simulink model "second_order_controllar"  (R2024b)
settings: Solver=FixedStepAuto  StartTime=0.0  StopTime=10.0  FixedStep=0.001  RelTol=1e-3
libraries: simulink x1
settings Model: Creator=elija  LastModifiedBy=elija

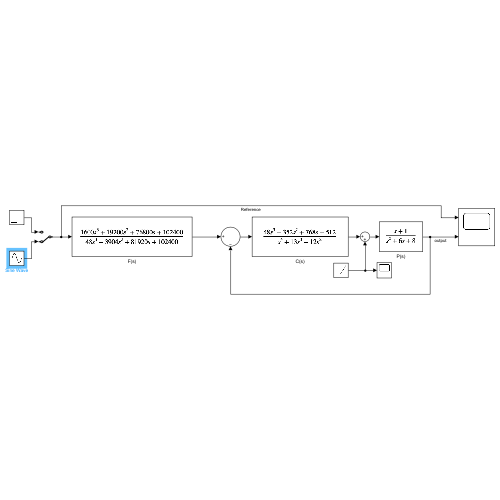
[thumbnail: Simulink's stored preview of the top-level diagram]
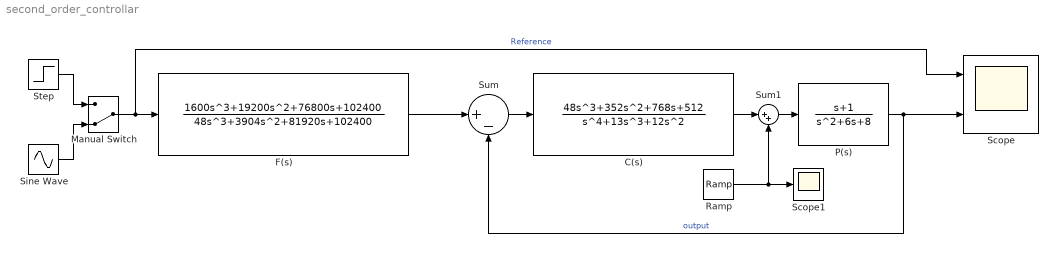
== system second_order_controllar ==
  C(s) : TransferFcn  Numerator=[48 352 768 512]  Denominator=[1 13 12 0 0]
  F(s) : TransferFcn  Numerator=[1600 19200 76800 102400]  Denominator=[48 3904 81920 102400]
  Manual Switch : ManualSwitch  CurrentSetting=0
  P(s) : TransferFcn  Numerator=[1 1]  Denominator=[1 6 8]
  Ramp : simulink/Sources/Ramp  slope=1  start=0  InitialOutput=0
  Scope : Scope  NumInputPorts=2
  Scope1 : Scope
  Sine Wave : Sin  Frequency=15  SampleTime=0
  Step : Step  SampleTime=0
  Sum : Sum  Inputs=|+-
  Sum1 : Sum  Inputs=|++
  wires:
  Step/1 -> Manual Switch/1
  F(s)/1 -> Sum/1
  Sum/1 -> C(s)/1
  C(s)/1 -> Sum1/1
  P(s)/1 -> Sum/2, Scope/2  "output"
  Sum1/1 -> P(s)/1
  Ramp/1 -> Scope1/1, Sum1/2
  Manual Switch/1 -> Scope/1, F(s)/1  "Reference"
  Sine Wave/1 -> Manual Switch/2
